simulink model "modelo_fibonacci"  (R2023b)
settings: Solver=FixedStepDiscrete  StartTime=0  StopTime=5  FixedStep=1  RelTol=1e-3
undefined symbols (not defined in the file): F0, F1
settings Model: Creator=alfre  LastModifiedBy=alfre

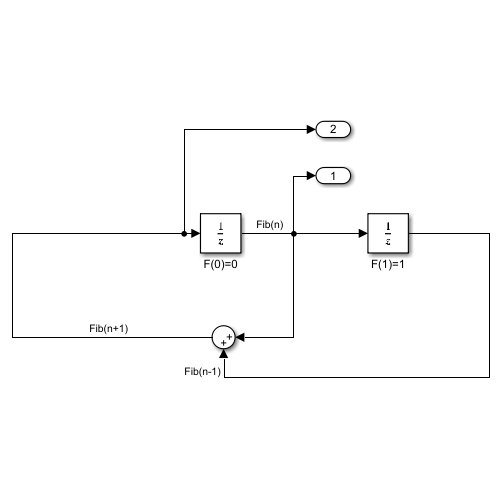
[thumbnail: Simulink's stored preview of the top-level diagram]
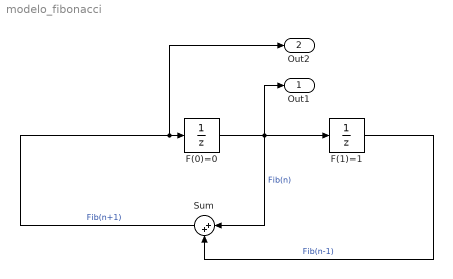
== system modelo_fibonacci ==
  F(0)=0 : UnitDelay  InitialCondition=F0  SampleTime=-1  HasFrameUpgradeWarning=on
  F(1)=1 : UnitDelay  InitialCondition=F1  SampleTime=-1  HasFrameUpgradeWarning=on
  Sum : Sum  Inputs=|++
  Out1 : Outport
  Out2 : Outport  Port=2
  wires:
  Sum/1 -> Out2/1, F(0)=0/1  "Fib(n+1)"
  F(0)=0/1 -> Out1/1, Sum/1, F(1)=1/1  "Fib(n)"
  F(1)=1/1 -> Sum/2  "Fib(n-1)"
